simulink model "Aktive_Schwingungsdaempfung_Simu"  (R2016a)
settings: Solver=VariableStepAuto  StartTime=0.0  StopTime=5  MaxStep=0.01  RelTol=1e-3
libraries: simulink x1
settings Model: Creator=Zehra Fatih  LastModifiedBy=Zehra Fatih

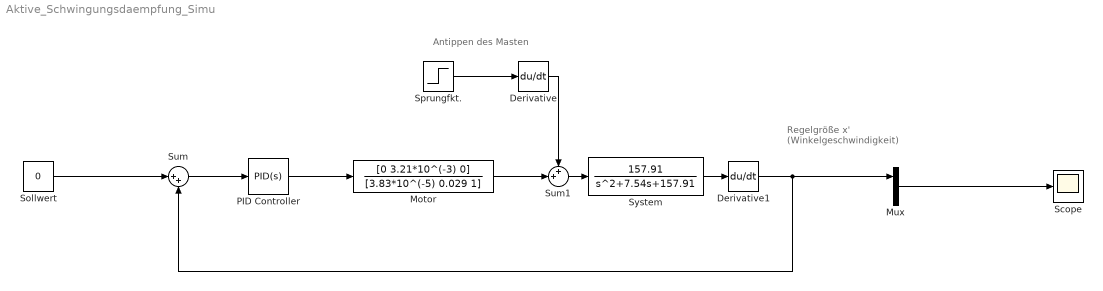
== system Aktive_Schwingungsdaempfung_Simu ==
  note: Antippen des Masten
  note: Regelgröße x'
      | (Winkelgeschwindigkeit)
  Derivative : Derivative
  Derivative1 : Derivative
  Motor : TransferFcn  Numerator=[0 3.21*10^(-3) 0]  Denominator=[3.83*10^(-5) 0.029 1]
  Mux : Mux  Inputs=2
  PID Controller : simulink/Continuous/PID Controller  Controller=PID  TimeDomain=Continuous-time  SampleTime=-1  IntegratorMethod=Forward Euler  FilterMethod=Forward Euler  Form=Parallel  UseFilter=on  ControllerParametersSource=internal  P=-3  I=0  D=0  N=100  InitialConditionSource=internal  InitialConditionForIntegrator=0  InitialConditionForFilter=0  ExternalReset=none  LimitOutput=off  UpperSaturationLimit=inf  LowerSaturationLimit=-inf  LinearizeAsGain=on  AntiWindupMode=none  Kb=1  TrackingMode=off  Kt=1  PParamMin=[]  PParamMax=[]  IParamMin=[]  IParamMax=[]  DParamMin=[]  DParamMax=[]  NParamMin=[]  NParamMax=[]  KbParamMin=[]  KbParamMax=[]  KtParamMin=[]  KtParamMax=[]  POutMin=[]  POutMax=[]  IOutMin=[]  IOutMax=[]  DOutMin=[]  DOutMax=[]  NOutMin=[]  NOutMax=[]  KbOutMin=[]  KbOutMax=[]  KtOutMin=[]  KtOutMax=[]  IntegratorOutMin=[]  IntegratorOutMax=[]  FilterOutMin=[]  FilterOutMax=[]  SumOutMin=[]  SumOutMax=[]  SumI1OutMin=[]  SumI1OutMax=[]  SumI2OutMin=[]  SumI2OutMax=[]  SumI3OutMin=[]  SumI3OutMax=[]  SumDOutMin=[]  SumDOutMax=[]  SaturationOutMin=[]  SaturationOutMax=[]  IntegratorContinuousStateAttributes=''  IntegratorStateMustResolveToSignalObject=off  IntegratorRTWStateStorageClass=Auto  FilterContinuousStateAttributes=''  FilterStateMustResolveToSignalObject=off  FilterRTWStateStorageClass=Auto  DifferentiatorICPrevScaledInput=0  DifferentiatorOutMin=[]  DifferentiatorOutMax=[]
  Scope : Scope
  Sollwert : Constant  Value=0
  Sprungfkt. : Step  After=-5  SampleTime=0
  Sum : Sum  Inputs=|++
  Sum1 : Sum  Inputs=++|
  System : TransferFcn  Numerator=[157.91]  Denominator=[1 7.54 157.91]
  wires:
  Sollwert/1 -> Sum/1
  Sum/1 -> PID Controller/1
  Sum1/1 -> System/1
  Mux/1 -> Scope/1
  Sprungfkt./1 -> Derivative/1
  Derivative/1 -> Sum1/1
  Motor/1 -> Sum1/2
  System/1 -> Derivative1/1
  PID Controller/1 -> Motor/1
  Derivative1/1 -> Sum/2, Mux/1
